simulink model "volt_sfunc"  (R2019a)
settings: Solver=VariableStepAuto  StartTime=0.0  StopTime=5  RelTol=1e-3
settings Model: Creator=USER  LastModifiedBy=USER

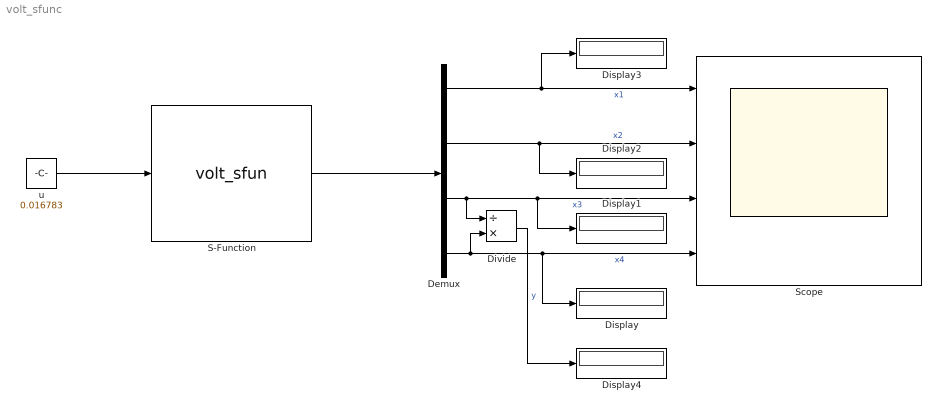
== system volt_sfunc ==
  Demux : Demux
  Display{,1..4} (5 alike) : Display
  Divide : Product  Inputs=/*
  S-Function : S-Function  FunctionName=volt_sfun  SFunctionDeploymentMode=off  EnableBusSupport=off
  Scope : Scope  NumInputPorts=4
  u : Constant  Value=0.016783
  wires:
  S-Function/1 -> Demux/1
  u/1 -> S-Function/1
  Demux/1 -> Display3/1, Scope/1  "x1"
  Demux/4 -> Divide/2, Display/1, Scope/4  "x4"
  Demux/3 -> Divide/1, Display1/1, Scope/3  "x3"
  Demux/2 -> Display2/1, Scope/2  "x2"
  Divide/1 -> Display4/1  "y"
